simulink model "ClimateControlSystemBlock"  (R2026a)
settings: Solver=VariableStepAuto
undefined symbols (not defined in the file): DiscIntNeverNeededParam
settings Model: Creator=nxg02009  LastModifiedBy=nxg02009

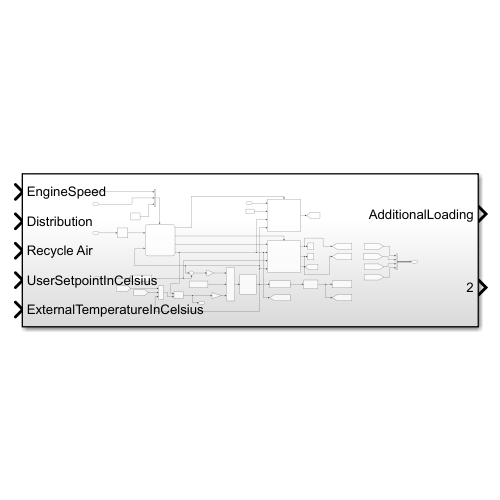
[thumbnail: Simulink's stored preview of the top-level diagram]
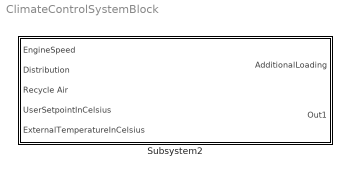
== system ClimateControlSystemBlock ==
  Subsystem2 : Subsystem

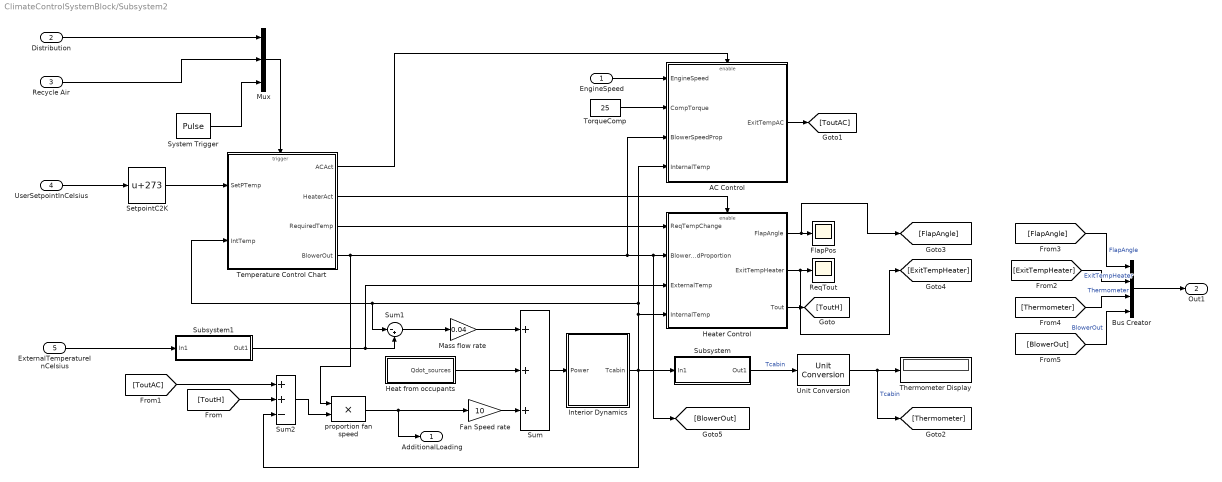
== system ClimateControlSystemBlock/Subsystem2 ==
  EngineSpeed : Inport  OutDataTypeStr=double  PortDimensions=1
  Distribution : Inport  Port=2  OutDataTypeStr=double
  Recycle Air : Inport  Port=3  OutDataTypeStr=double
  UserSetpointInCelsius : Inport  Port=4
  ExternalTemperatureInCelsius : Inport  Port=5
  AC Control : Subsystem  TreatAsAtomicUnit=on
  Bus Creator : BusCreator  Inputs=4  OutDataTypeStr=Bus: OutputBus
  Fan Speed rate : Gain  Gain=10  SaturateOnIntegerOverflow=on  OutDataTypeStr=Inherit: Same as input  ParamDataTypeStr=Inherit: Same as input
  FlapPos : Scope
      settings: ActiveDisplayYMinimum=-1  ActiveDisplayYMaximum=1
  Heat from occupants : Subsystem  mask(Heat from occupants){N=3}
      mask prompts: N "Number of occupants:"
      settings: AttributesFormatString=No. of occupants: %<N>
      mask Display: disp('Heat Sources')
  Heater Control : Subsystem  TreatAsAtomicUnit=on
  Interior Dynamics : Subsystem  mask(Vehicle Cabin Dynamics){}
      mask Display: image('$imagefile') % use "Edit Image" on toolstrip to change
  Mass flow rate : Gain  Gain=0.04  SaturateOnIntegerOverflow=on  OutDataTypeStr=Inherit: Same as input  ParamDataTypeStr=Inherit: Same as input
  Mux : Mux  Inputs=3
  ReqTout : Scope
      settings: ActiveDisplayYMinimum=-1  ActiveDisplayYMaximum=1
  SetpointC2K : Bias  Bias=273  SaturateOnIntegerOverflow=off
  Subsystem : Subsystem
      mask Display: disp('Kelvin to Celsius')
  Subsystem1 : Subsystem
      mask Display: disp('Celsius to Kelvin')
  Sum : Sum  Inputs=+++  InputSameDT=on  SaturateOnIntegerOverflow=on  OutDataTypeStr=Inherit: Same as first input
  Sum1 : Sum  Inputs=|-+  InputSameDT=on  SaturateOnIntegerOverflow=on  OutDataTypeStr=Inherit: Same as first input
  Sum2 : Sum  Inputs=++-  InputSameDT=on  SaturateOnIntegerOverflow=on  OutDataTypeStr=Inherit: Same as first input
  System Trigger : DiscretePulseGenerator  SampleTime=-1
  Temperature Control Chart : Stateflow chart  TreatAsAtomicUnit=on
  Thermometer Display : Display
  TorqueComp : Constant  Value=25
  Unit Conversion : UnitConversion
  proportion fan speed : Product  InputSameDT=on  SaturateOnIntegerOverflow=on  OutDataTypeStr=Inherit: Same as first input
  AdditionalLoading : Outport  OutDataTypeStr=double  PortDimensions=1  VectorParamsAs1DForOutWhenUnconnected=off
  Out1 : Outport  Port=2  OutDataTypeStr=Bus: OutputBus
  wires:
  AC Control/1(ExitTempAC) -> [ToutAC]
  [BlowerOut] -> Bus Creator/4  "BlowerOut"
  Interior Dynamics/1("Tcabin ") -> Heater Control/4(InternalTemp), Temperature Control Chart/2(IntTemp), Sum1/1, AC Control/4(InternalTemp), Sum2/3, Subsystem/1(In1)
  TorqueComp/1 -> AC Control/2(CompTorque)
  proportion fan speed/1 -> AdditionalLoading/1, Fan Speed rate/1
  Heater Control/2(ExitTempHeater) -> [ExitTempHeater], ReqTout/1
  [Thermometer] -> Bus Creator/3  "Thermometer"
  EngineSpeed/1 -> AC Control/1(EngineSpeed)
  Heater Control/3(Tout) -> [ToutH]
  Fan Speed rate/1 -> Sum/3
  Sum/1 -> Interior Dynamics/1(Power)
  Recycle Air/1 -> Mux/2
  Sum1/1 -> Mass flow rate/1
  Subsystem/1(Out1) -> Unit Conversion/1  "Tcabin"
  SetpointC2K/1 -> Temperature Control Chart/1(SetPTemp)
  Heater Control/1(FlapAngle) -> [FlapAngle], FlapPos/1
  Sum2/1 -> proportion fan speed/2
  Unit Conversion/1 -> [Thermometer], Thermometer Display/1  "Tcabin"
  Temperature Control Chart/3(RequiredTemp) -> Heater Control/1(ReqTempChange)
  [ToutH] -> Sum2/2
  Subsystem1/1(Out1) -> Heater Control/3(ExternalTemp), Sum1/2
  [ExitTempHeater] -> Bus Creator/2  "ExitTempHeater"
  Distribution/1 -> Mux/1
  Bus Creator/1 -> Out1/1
  Temperature Control Chart/4(BlowerOut) -> [BlowerOut], Heater Control/2(BlowerSpeedProportion), AC Control/3(BlowerSpeedProp), proportion fan speed/1
  ExternalTemperatureInCelsius/1 -> Subsystem1/1(In1)
  Temperature Control Chart/1(" ACAct") -> AC Control/Enable
  Mass flow rate/1 -> Sum/1
  Mux/1 -> Temperature Control Chart/Trigger
  UserSetpointInCelsius/1 -> SetpointC2K/1
  Heat from occupants/1(Qdot_sources) -> Sum/2
  [ToutAC] -> Sum2/1
  System Trigger/1 -> Mux/3
  [FlapAngle] -> Bus Creator/1  "FlapAngle"
  Temperature Control Chart/2(" HeaterAct") -> Heater Control/Enable

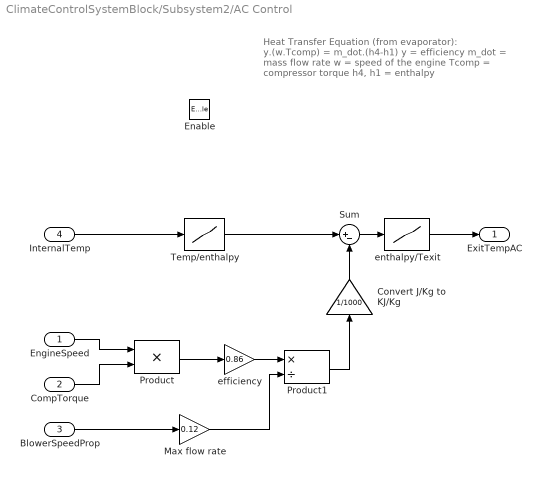
== system ClimateControlSystemBlock/Subsystem2/AC Control ==
  note: Heat Transfer Equation (from evaporator):
      |
      | y.(w.Tcomp) = m_dot.(h4-h1)
      |
      | y = efficiency
      | m_dot = mass flow rate
      | w = speed of the engine
      | Tcomp = compressor torque
      | h4, h1 = enthalpy
  EngineSpeed : Inport
  CompTorque : Inport  Port=2
  BlowerSpeedProp : Inport  Port=3
  InternalTemp : Inport  Port=4
  Enable : EnablePort  StatesWhenEnabling=reset  PropagateVarSize=During execution  ZeroCross=off
  Convert J/Kg to KJ/Kg : Gain  Gain=1/1000
  Max flow rate : Gain  Gain=0.12  SaturateOnIntegerOverflow=on  OutDataTypeStr=Inherit: Same as input  ParamDataTypeStr=Inherit: Same as input
  Product : Product  InputSameDT=on  SaturateOnIntegerOverflow=on  OutDataTypeStr=Inherit: Same as first input
  Product1 : Product  Inputs=*/  InputSameDT=on  SaturateOnIntegerOverflow=on  OutDataTypeStr=Inherit: Same as first input
  Sum : Sum  Inputs=|+-  InputSameDT=on  SaturateOnIntegerOverflow=on  OutDataTypeStr=Inherit: Same as first input
  Temp/enthalpy : Lookup_n-D  NumberOfTableDimensions=1  BreakpointsForDimension1=[220 230 240 250 260 270 280 285 290 295 300 305 310 315 320]  Table=[219.97 230.02 240.02 250.05 260.09 270.11 280.13 285.14 290.16 295.17 300.19 305.22 310.24 315.27 320.29]  SaturateOnIntegerOverflow=on
  efficiency : Gain  Gain=0.86  SaturateOnIntegerOverflow=on  OutDataTypeStr=Inherit: Same as input  ParamDataTypeStr=Inherit: Same as input
  enthalpy/Texit : Lookup_n-D  NumberOfTableDimensions=1  BreakpointsForDimension1=[219.97 230.02 240.02 250.05 260.09 270.11 280.13 285.14 290.16 295.17 300.19 305.22 310.24 315.27 320.29]  Table=[220 230 240 250 260 270 280 285 290 295 300 305 310 315 320]  SaturateOnIntegerOverflow=on
  ExitTempAC : Outport  OutputWhenDisabled=reset  InitialOutput=0  VectorParamsAs1DForOutWhenUnconnected=off
  wires:
  Convert J/Kg to KJ/Kg/1 -> Sum/2
  Sum/1 -> enthalpy/Texit/1
  Product1/1 -> Convert J/Kg to KJ/Kg/1
  Temp/enthalpy/1 -> Sum/1
  InternalTemp/1 -> Temp/enthalpy/1
  enthalpy/Texit/1 -> ExitTempAC/1
  Max flow rate/1 -> Product1/2
  BlowerSpeedProp/1 -> Max flow rate/1
  efficiency/1 -> Product1/1
  Product/1 -> efficiency/1
  CompTorque/1 -> Product/2
  EngineSpeed/1 -> Product/1

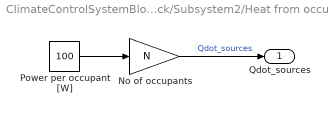
== system ClimateControlSystemBlock/Subsystem2/Heat from occupants ==
  No of occupants : Gain  Gain=N  SaturateOnIntegerOverflow=on  OutDataTypeStr=Inherit: Same as input  ParamDataTypeStr=Inherit: Same as input
  Power per occupant [W] : Constant  Value=100
  Qdot_sources : Outport  VectorParamsAs1DForOutWhenUnconnected=off
  wires:
  Power per occupant [W]/1 -> No of occupants/1
  No of occupants/1 -> Qdot_sources/1  "Qdot_sources"

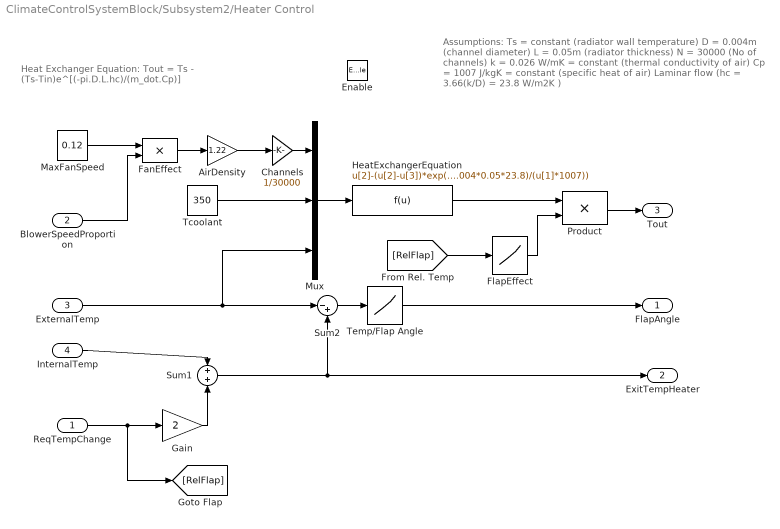
== system ClimateControlSystemBlock/Subsystem2/Heater Control ==
  note: Assumptions:
      | Ts = constant (radiator wall temperature)
      | D = 0.004m (channel diameter)
      | L = 0.05m (radiator thickness)
      | N = 30000 (No of channels)
      |
      | k = 0.026 W/mK = constant (thermal conductivity of air)
      | Cp = 1007 J/kgK = constant (specific heat of air)
      | Laminar flow (hc = 3.66(k/D) = 23.8 W/m2K )
  note: Heat Exchanger Equation:
      | Tout = Ts - (Ts-Tin)e^[(-pi.D.L.hc)/(m_dot.Cp)]
  ReqTempChange : Inport
  BlowerSpeedProportion : Inport  Port=2
  ExternalTemp : Inport  Port=3
  InternalTemp : Inport  Port=4
  Enable : EnablePort  StatesWhenEnabling=reset  PropagateVarSize=During execution  ZeroCross=off
  AirDensity : Gain  Gain=1.22  SaturateOnIntegerOverflow=on  OutDataTypeStr=Inherit: Same as input  ParamDataTypeStr=Inherit: Same as input
  Channels : Gain  Gain=1/30000  SaturateOnIntegerOverflow=on  OutDataTypeStr=Inherit: Same as input  ParamDataTypeStr=Inherit: Same as input
  FanEffect : Product  InputSameDT=on  SaturateOnIntegerOverflow=on  OutDataTypeStr=Inherit: Same as first input
  FlapEffect : Lookup_n-D  NumberOfTableDimensions=1  BreakpointsForDimension1="[0 3 5 10 50  90 100 200 ]"  Table="[0 300 100  10 10  10 3 1]"  SaturateOnIntegerOverflow=on
  Gain : Gain  Gain=2  SaturateOnIntegerOverflow=on  OutDataTypeStr=Inherit: Same as input  ParamDataTypeStr=Inherit: Same as input
  HeatExchangerEquation : Fcn  Expr=u[2]-(u[2]-u[3])*exp(-(pi*0.004*0.05*23.8)/(u[1]*1007))
  MaxFanSpeed : Constant  Value=0.12
  Mux : Mux  Inputs=3
  Product : Product  InputSameDT=on  SaturateOnIntegerOverflow=on  OutDataTypeStr=Inherit: Same as first input
  Sum1 : Sum  InputSameDT=on  SaturateOnIntegerOverflow=on  OutDataTypeStr=Inherit: Same as first input
  Sum2 : Sum  Inputs=|-+  InputSameDT=on  SaturateOnIntegerOverflow=on  OutDataTypeStr=Inherit: Same as first input
  "Tcoolant " : Constant  Value=350
  Temp/Flap Angle : Lookup_n-D  NumberOfTableDimensions=1  BreakpointsForDimension1=[0 10 20 30 40 50 60 75 100 200]  Table=[0 20 30 45 60 75 90 90 90 90]  SaturateOnIntegerOverflow=on
  FlapAngle : Outport  OutputWhenDisabled=reset  InitialOutput=0  VectorParamsAs1DForOutWhenUnconnected=off
  ExitTempHeater : Outport  Port=2  OutputWhenDisabled=reset  InitialOutput=0  VectorParamsAs1DForOutWhenUnconnected=off
  Tout : Outport  Port=3  OutputWhenDisabled=reset  InitialOutput=0  VectorParamsAs1DForOutWhenUnconnected=off
  wires:
  HeatExchangerEquation/1 -> Product/1
  ExternalTemp/1 -> Mux/3, Sum2/1
  BlowerSpeedProportion/1 -> FanEffect/2
  MaxFanSpeed/1 -> FanEffect/1
  FanEffect/1 -> AirDensity/1
  Mux/1 -> HeatExchangerEquation/1
  AirDensity/1 -> Channels/1
  Channels/1 -> Mux/1
  "Tcoolant "/1 -> Mux/2
  Product/1 -> Tout/1
  Temp/Flap Angle/1 -> FlapAngle/1
  Sum2/1 -> Temp/Flap Angle/1
  InternalTemp/1 -> Sum1/1
  Gain/1 -> Sum1/2
  Sum1/1 -> ExitTempHeater/1, Sum2/2
  ReqTempChange/1 -> Gain/1, [RelFlap]
  FlapEffect/1 -> Product/2
  [RelFlap] -> FlapEffect/1

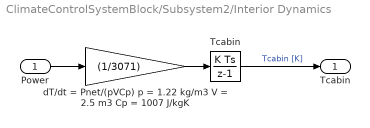
== system ClimateControlSystemBlock/Subsystem2/Interior Dynamics ==
  Power : Inport
  Tcabin : DiscreteIntegrator  InitialCondition=273+29  SampleTime=-1  ICPrevOutput=DiscIntNeverNeededParam  ICPrevScaledInput=DiscIntNeverNeededParam
  dT/dt = Pnet/(pVCp) p = 1.22 kg/m3 V = 2.5 m3 Cp = 1007 J/kgK : Gain  Gain=(1/3071)  SaturateOnIntegerOverflow=on  OutDataTypeStr=Inherit: Same as input  ParamDataTypeStr=Inherit: Same as input
  "Tcabin " : Outport  VectorParamsAs1DForOutWhenUnconnected=off
  wires:
  Power/1 -> dT/dt = Pnet/(pVCp) p = 1.22 kg/m3 V = 2.5 m3 Cp = 1007 J/kgK/1
  dT/dt = Pnet/(pVCp) p = 1.22 kg/m3 V = 2.5 m3 Cp = 1007 J/kgK/1 -> Tcabin/1
  Tcabin/1 -> "Tcabin "/1  "Tcabin [K]"

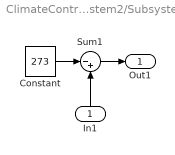
== system ClimateControlSystemBlock/Subsystem2/Subsystem ==
  In1 : Inport
  Constant : Constant  Value=273
  Sum1 : Sum  Inputs=|-+  InputSameDT=on  SaturateOnIntegerOverflow=on  OutDataTypeStr=Inherit: Same as first input
  Out1 : Outport  VectorParamsAs1DForOutWhenUnconnected=off
  wires:
  Sum1/1 -> Out1/1
  In1/1 -> Sum1/2
  Constant/1 -> Sum1/1

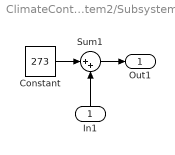
== system ClimateControlSystemBlock/Subsystem2/Subsystem1 ==
  In1 : Inport
  Constant : Constant  Value=273
  Sum1 : Sum  Inputs=|++  InputSameDT=on  SaturateOnIntegerOverflow=on  OutDataTypeStr=Inherit: Same as first input
  Out1 : Outport  VectorParamsAs1DForOutWhenUnconnected=off
  wires:
  Constant/1 -> Sum1/1
  In1/1 -> Sum1/2
  Sum1/1 -> Out1/1

== stateflow chart ClimateControlSystemBlock/Subsystem2/Temperature Control Chart ==
  state Blower [parallel]
    during:setpoint_calc();
    settings: executionOrder=1
    state Blower_off
      entry:BlowerOut=0.0;
    state Blower_on
      state Blower_1
        entry:BlowerOut=0.2;
      state Blower_2
        entry:BlowerOut=0.4;
      state Blower_3
        entry:BlowerOut=0.6;
      state Blower_4
        entry:BlowerOut=0.8;
      state Blower_5
        entry:BlowerOut=1.0;
      (default) -> Blower_1
      Blower_on -> Blower_1 [order 5] : E[~in(Blower_1) && in_temp_range(1.5,5)]
      Blower_on -> Blower_2 [order 4] : E[~in(Blower_2) && in_temp_range(7,10)]
      Blower_on -> Blower_3 [order 3] : E[~in(Blower_3) && in_temp_range(12,15)]
      Blower_on -> Blower_4 [order 2] : E[~in(Blower_4) && in_temp_range(17,20)]
      Blower_on -> Blower_5 [order 1] : E[~in(Blower_5) && in_temp_range(22,200)]
    state setpoint_calc() [function]
      (default) -> (junction 51) : {RequiredTemp = SetPTemp-IntTemp;}
      (junction 51) -> (junction 48) [order 1] : [RequiredTemp<0.0]
          | {absTempDiff = -RequiredTemp;}
      (junction 51) -> (junction 49) [order 2] : {absTempDiff = RequiredTemp;}
    state b = in_temp_range(minTemp,maxTemp) [function]
      (default) -> (junction 50) : {b = (absTempDiff>minTemp) &&  ...
          |         (absTempDiff<maxTemp);}
    (default) -> Blower_off
    Blower_off -> Blower_on : E[absTempDiff<203 || absTempDiff>1]
    Blower_on -> Blower_off [order 1] : E[absTempDiff>203 || absTempDiff<=eps]
  state Heater_AC [parallel]
    settings: executionOrder=2
    state H_offAC_off
    state ACAct
    state HeaterAct
    ACAct -> H_offAC_off : E[SetPTemp-IntTemp>=-0.5]
    HeaterAct -> H_offAC_off : E[SetPTemp-IntTemp<=0.5]
    H_offAC_off -> HeaterAct [order 2] : E[SetPTemp-IntTemp>0.55]
    H_offAC_off -> ACAct [order 1] : E[SetPTemp-IntTemp<-0.55]
    (default) -> H_offAC_off
  state AirDist [parallel]
    settings: executionOrder=3
    state Feet
    state Face
    state Defrost
    (default) -> Face
    Feet -> Defrost : DistReq
    Face -> Feet : DistReq
    Defrost -> Face : DistReq
  state Recyc_Air [parallel]
    settings: executionOrder=4
    state Recyc_on
    state Recyc_off
    (default) -> Recyc_on
    Recyc_on -> Recyc_off [order 2] : RecycReq
    Recyc_off -> Recyc_on : RecycReq
    Recyc_on -> Recyc_off [order 1] : en(AirDist.Defrost)
  data: minTemp function_input double; b function_output boolean; maxTemp function_input double; ACAct output boolean; SetPTemp input double; IntTemp input double; HeaterAct output boolean; RequiredTemp output double; BlowerOut output double; absTempDiff local double
  events: DistReq input EITHER_EDGE_EVENT; RecycReq input EITHER_EDGE_EVENT; E input EITHER_EDGE_EVENT
